simulink model "nolineal_closeloop_referencia"  (R2014a)
settings: Solver=ode15s  StartTime=0.0  StopTime=900  RelTol=1e-3
libraries: simulink x1
settings Model: Creator=JuanPablo  LastModifiedBy=juanr
settings DataIOCC: SignalLoggingSaveFormat=ModelDataLogs
settings OptimizationCC: ExpressionDepthLimit=2147483647
settings DebuggingCC: AlgebraicLoopMsg=none  UnderspecifiedInitializationDetection=Classic  SolverPrmCheckMsg=none  FcnCallInpInsideContextMsg=EnableAllAsWarning  StateNameClashWarn=warning

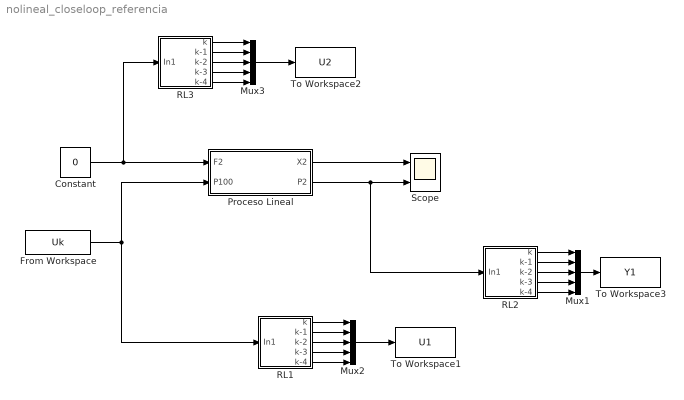
== system nolineal_closeloop_referencia ==
  Constant : Constant  Value=0
  From Workspace : FromWorkspace  VariableName=Uk  SampleTime=0
  Mux1 : Mux  Inputs=5
  Mux2 : Mux  Inputs=5
  Mux3 : Mux  Inputs=5
  Proceso Lineal : Subsystem  TreatAsAtomicUnit=on
  RL1 : Subsystem  TreatAsAtomicUnit=on
  RL2 : Subsystem  TreatAsAtomicUnit=on
  RL3 : Subsystem  TreatAsAtomicUnit=on
  Scope : Scope  NumInputPorts=2
      settings: TimeRange=450  YMin=-1~-0.05  YMax=1~0.3  SaveName=openloop
  To Workspace1 : ToWorkspace  VariableName=U1  SaveFormat=Timeseries  SampleTime=5
  To Workspace2 : ToWorkspace  VariableName=U2  SaveFormat=Timeseries  SampleTime=5
  To Workspace3 : ToWorkspace  VariableName=Y1  SaveFormat=Timeseries  SampleTime=5
  wires:
  Proceso Lineal/1(X2) -> Scope/1
  Constant/1 -> RL3/1(In1), Proceso Lineal/1("F2 ")
  RL1/1(k) -> Mux2/1
  RL1/2(k-1) -> Mux2/2
  RL1/3(k-2) -> Mux2/3
  Mux2/1 -> To Workspace1/1
  From Workspace/1 -> RL1/1(In1), Proceso Lineal/2(P100)
  RL1/4(k-3) -> Mux2/4
  RL1/5(k-4) -> Mux2/5
  RL2/1(k) -> Mux1/1
  RL2/2(k-1) -> Mux1/2
  RL2/3(k-2) -> Mux1/3
  Mux1/1 -> To Workspace3/1
  Proceso Lineal/2(P2) -> RL2/1(In1), Scope/2
  RL2/4(k-3) -> Mux1/4
  RL2/5(k-4) -> Mux1/5
  Mux3/1 -> To Workspace2/1
  RL3/1(k) -> Mux3/1
  RL3/5(k-4) -> Mux3/5
  RL3/3(k-2) -> Mux3/3
  RL3/4(k-3) -> Mux3/4
  RL3/2(k-1) -> Mux3/2

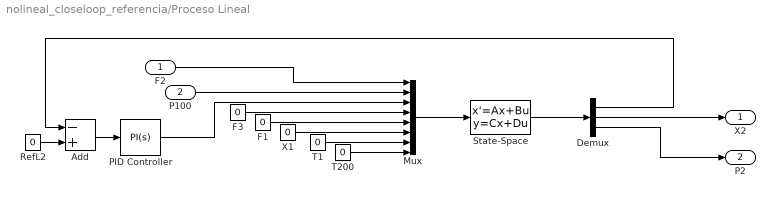
== system nolineal_closeloop_referencia/Proceso Lineal ==
  "F2 " : Inport
  P100 : Inport  Port=2
  Add : Sum  Inputs=-+
  Demux : Demux  Outputs=3
  F1 : Constant  Value=0
  F3 : Constant  Value=0
  Mux : Mux  Inputs=8
  PID Controller : simulink/Continuous/PID Controller  Controller=PI  TimeDomain=Continuous-time  SampleTime=1  IntegratorMethod=Forward Euler  FilterMethod=Forward Euler  Form=Parallel  P=-0.601  I=-0.601/92.671  D=0  N=100  InitialConditionSource=internal  InitialConditionForIntegrator=0  InitialConditionForFilter=0  ExternalReset=none  LimitOutput=off  UpperSaturationLimit=inf  LowerSaturationLimit=-inf  LinearizeAsGain=on  AntiWindupMode=none  Kb=1  TrackingMode=off  Kt=1  PParamMin=[]  PParamMax=[]  IParamMin=[]  IParamMax=[]  DParamMin=[]  DParamMax=[]  NParamMin=[]  NParamMax=[]  KbParamMin=[]  KbParamMax=[]  KtParamMin=[]  KtParamMax=[]  POutMin=[]  POutMax=[]  IOutMin=[]  IOutMax=[]  DOutMin=[]  DOutMax=[]  NOutMin=[]  NOutMax=[]  KbOutMin=[]  KbOutMax=[]  KtOutMin=[]  KtOutMax=[]  IntegratorOutMin=[]  IntegratorOutMax=[]  FilterOutMin=[]  FilterOutMax=[]  SumOutMin=[]  SumOutMax=[]  SumI1OutMin=[]  SumI1OutMax=[]  SumI2OutMin=[]  SumI2OutMax=[]  SumI3OutMin=[]  SumI3OutMax=[]  SumDOutMin=[]  SumDOutMax=[]  SaturationOutMin=[]  SaturationOutMax=[]  IntegratorContinuousStateAttributes=''  IntegratorStateMustResolveToSignalObject=off  IntegratorRTWStateStorageClass=Auto  FilterContinuousStateAttributes=''  FilterStateMustResolveToSignalObject=off  FilterRTWStateStorageClass=Auto
  "RefL2 " : Constant  Value=0
  State-Space : StateSpace  A=[0 0.10455 0.37935; 0 -0.1 0; 0 -0.10340e-1 -0.54738e-1]  B=[-0.1 -0.37266 0 -0.36676 0.38605 0 -0.3636e-1 0; -0.1 0 0 0 0.1 0.1 0 0; 0 0.36914e-1 -0.75272e-2 0.36302e-1 0.32268e-2 0 0.35972e-2 0.17785e-1]  C=[1 0 0; 0 1 0; 0 0 1]  D=zeros(3,8)  X0=0
  T1 : Constant  Value=0
  T200 : Constant  Value=0
  X1 : Constant  Value=0
  X2 : Outport
  P2 : Outport  Port=2
  wires:
  Mux/1 -> State-Space/1
  State-Space/1 -> Demux/1
  "F2 "/1 -> Mux/1
  P100/1 -> Mux/2
  PID Controller/1 -> Mux/3
  F3/1 -> Mux/4
  F1/1 -> Mux/5
  X1/1 -> Mux/6
  T1/1 -> Mux/7
  T200/1 -> Mux/8
  Demux/1 -> Add/1
  Demux/2 -> X2/1
  Demux/3 -> P2/1
  Add/1 -> PID Controller/1
  "RefL2 "/1 -> Add/2

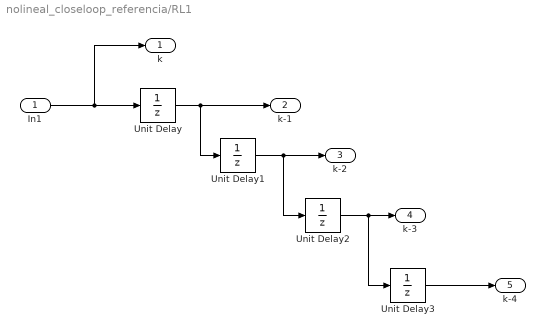
== system nolineal_closeloop_referencia/RL1 ==
  In1 : Inport
  Unit Delay{,1..3} (4 alike) : UnitDelay  SampleTime=5
  k : Outport
  k-1 : Outport  Port=2
  k-2 : Outport  Port=3
  k-3 : Outport  Port=4
  k-4 : Outport  Port=5
  wires:
  In1/1 -> k/1, Unit Delay/1
  Unit Delay/1 -> Unit Delay1/1, k-1/1
  Unit Delay1/1 -> Unit Delay2/1, k-2/1
  Unit Delay2/1 -> Unit Delay3/1, k-3/1
  Unit Delay3/1 -> k-4/1

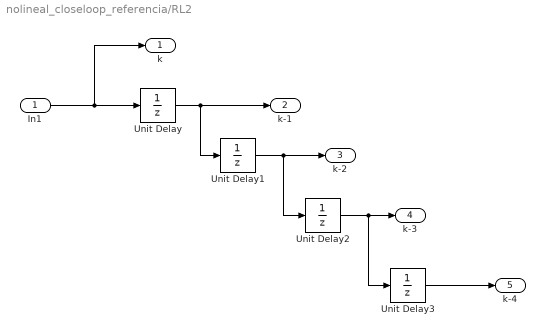
== system nolineal_closeloop_referencia/RL2 ==
  In1 : Inport
  Unit Delay{,1..3} (4 alike) : UnitDelay  SampleTime=5
  k : Outport
  k-1 : Outport  Port=2
  k-2 : Outport  Port=3
  k-3 : Outport  Port=4
  k-4 : Outport  Port=5
  wires:
  In1/1 -> k/1, Unit Delay/1
  Unit Delay/1 -> Unit Delay1/1, k-1/1
  Unit Delay1/1 -> Unit Delay2/1, k-2/1
  Unit Delay2/1 -> Unit Delay3/1, k-3/1
  Unit Delay3/1 -> k-4/1

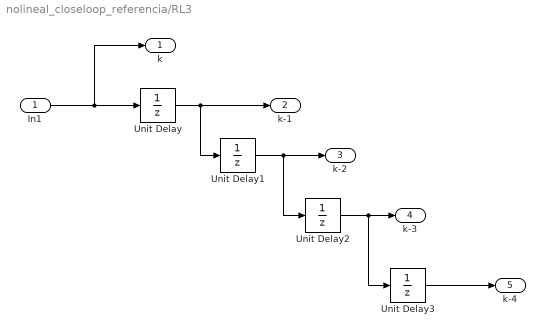
== system nolineal_closeloop_referencia/RL3 ==
  In1 : Inport
  Unit Delay{,1..3} (4 alike) : UnitDelay  SampleTime=5
  k : Outport
  k-1 : Outport  Port=2
  k-2 : Outport  Port=3
  k-3 : Outport  Port=4
  k-4 : Outport  Port=5
  wires:
  In1/1 -> k/1, Unit Delay/1
  Unit Delay/1 -> Unit Delay1/1, k-1/1
  Unit Delay1/1 -> Unit Delay2/1, k-2/1
  Unit Delay2/1 -> Unit Delay3/1, k-3/1
  Unit Delay3/1 -> k-4/1
